simulink model "myexp6_2"  (R2022a)
settings: Solver=VariableStepAuto  StartTime=0.0  StopTime=10000  RelTol=1e-3
values from neighbouring files (symbols this model uses):
  Ns = Ns_list(i)    [exp6_1.m]
libraries: commsink2 x9, commchan3 x4, commrandsrc3 x4, dspsigops x4, dspstat3 x2
settings Model: Creator=惠普  LastModifiedBy=惠普

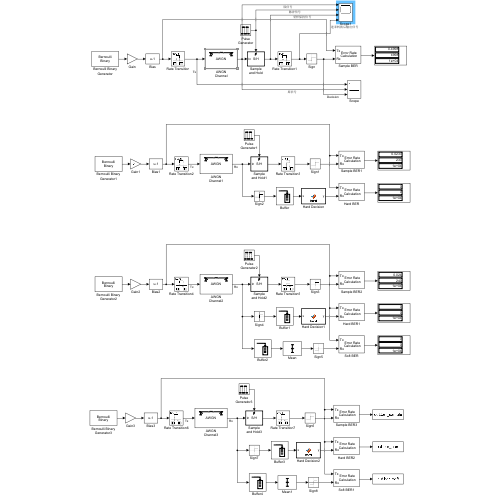
[thumbnail: Simulink's stored preview of the top-level diagram]
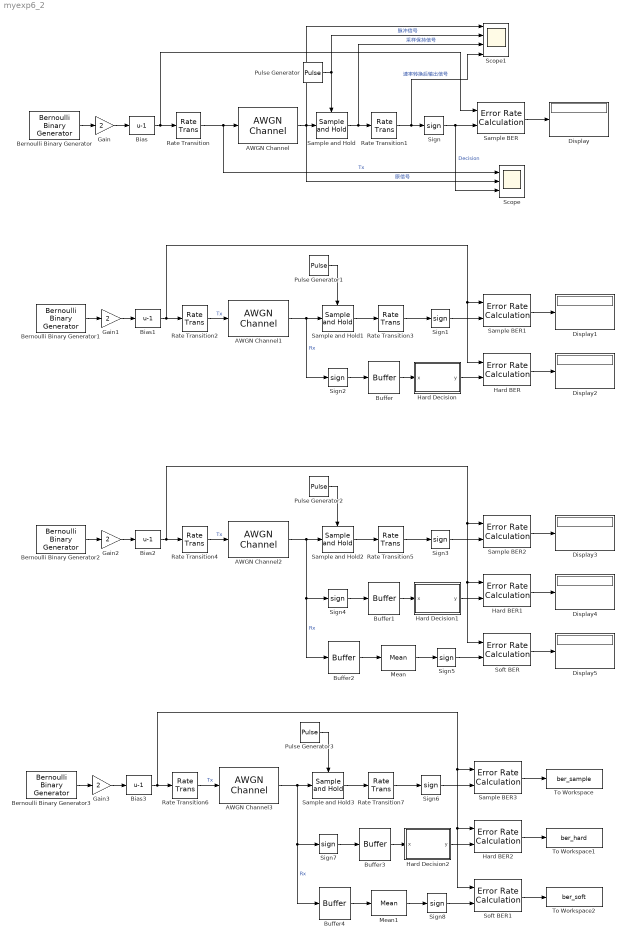
== system myexp6_2 ==
  AWGN Channel{,1..3} (4 alike) : commchan3/AWGN Channel  InputProcessing=Columns as channels (frame based)  seed=137  noiseMode=Variance from mask  EbNodB=10  EsNodB=10  SNRdB=10  bitsPerSym=1  Ps=1  Tsym=1  variance=sigma2
  Bernoulli Binary Generator{,1..3} (4 alike) : commrandsrc3/Bernoulli Binary Generator  ProbabilityOfZero=0.5  SeedSource=Auto  Seed=0  SampleTime=1  SamplesPerFrame=1  OutputDataType=double  SimulateUsing=Interpreted execution
  Bias{,1..3} (4 alike) : Bias  Bias=-1  SaturateOnIntegerOverflow=off
  Buffer{,1..4} (5 alike) : Buffer  N=Ns  OutputFrames=off
  Display{,1..5} (6 alike) : Display
  Gain{,1..3} (4 alike) : Gain  Gain=2
  Hard BER : commsink2/Error Rate Calculation  N=1  st_delay=0  cp_mode=Entire frame  subframe=[]  PMode=Port  WsName=ErrorVec  RsMode2=off  stop=off  numErr=100  maxBits=1e6
  Hard BER1 : commsink2/Error Rate Calculation  N=1  st_delay=0  cp_mode=Entire frame  subframe=[]  PMode=Port  WsName=ErrorVec  RsMode2=off  stop=off  numErr=100  maxBits=1e6
  Hard BER2 : commsink2/Error Rate Calculation  N=1  st_delay=0  cp_mode=Entire frame  subframe=[]  PMode=Port  WsName=ErrorVec  RsMode2=off  stop=off  numErr=100  maxBits=1e6
  Hard Decision : MATLAB Function  TreatAsAtomicUnit=on
  Hard Decision1 : MATLAB Function  TreatAsAtomicUnit=on
  Hard Decision2 : MATLAB Function  TreatAsAtomicUnit=on
  Mean : dspstat3/Mean  run=off  InputProcessing=Columns as channels (frame based)  reset_popup=None  directionMode=Each column  dimension=1  roiEnable=off  roiType=Rectangles  roiPortion=Entire ROI  roiOutput=Individual statistics for each ROI  roiFlag=off  roundingMode=Floor  overflowMode=off  outputDataTypeStr=Inherit: Same as accumulator  outputMin=[]  outputMax=[]  outputLastDataTypeStr=Inherit: Same as accumulator
  Mean1 : dspstat3/Mean  run=off  InputProcessing=Columns as channels (frame based)  reset_popup=None  directionMode=Each column  dimension=1  roiEnable=off  roiType=Rectangles  roiPortion=Entire ROI  roiOutput=Individual statistics for each ROI  roiFlag=off  roundingMode=Floor  overflowMode=off  outputDataTypeStr=Inherit: Same as accumulator  outputMin=[]  outputMax=[]  outputLastDataTypeStr=Inherit: Same as accumulator
  Pulse Generator : DiscretePulseGenerator  Period=Ns  PhaseDelay=5  SampleTime=1/Ns
  Pulse Generator1 : DiscretePulseGenerator  Period=Ns  SampleTime=1/Ns
  Pulse Generator2 : DiscretePulseGenerator  Period=Ns  SampleTime=1/Ns
  Pulse Generator3 : DiscretePulseGenerator  Period=Ns  SampleTime=1/Ns
  Rate Transition{,2,4,6} (4 alike) : RateTransition  Integrity=off  OutPortSampleTimeOpt=Multiple of input port sample time  OutPortSampleTimeMultiple=1/Ns
  Rate Transition{1,3,5,7} (4 alike) : RateTransition  OutPortSampleTimeOpt=Multiple of input port sample time  OutPortSampleTimeMultiple=Ns
  Sample and Hold{,1..3} (4 alike) : dspsigops/Sample and Hold  trig=Rising edge  initCond=0  latchinput=off
  Sample BER{,1..3} (4 alike) : commsink2/Error Rate Calculation  N=0  st_delay=0  cp_mode=Entire frame  subframe=[]  PMode=Port  WsName=ErrorVec  RsMode2=off  stop=off  numErr=100  maxBits=1e6
  Scope : Scope  NumInputPorts=3
  Scope1 : Scope  NumInputPorts=4
  Sign{,1..8} (9 alike) : Signum
  Soft BER : commsink2/Error Rate Calculation  N=1  st_delay=0  cp_mode=Entire frame  subframe=[]  PMode=Port  WsName=ErrorVec  RsMode2=off  stop=off  numErr=100  maxBits=1e6
  Soft BER1 : commsink2/Error Rate Calculation  N=1  st_delay=0  cp_mode=Entire frame  subframe=[]  PMode=Port  WsName=ErrorVec  RsMode2=off  stop=off  numErr=100  maxBits=1e6
  To Workspace : ToWorkspace  VariableName=ber_sample  SampleTime=-1
      settings: MaxDataPoints=1
  To Workspace1 : ToWorkspace  VariableName=ber_hard  SampleTime=-1
      settings: MaxDataPoints=1
  To Workspace2 : ToWorkspace  VariableName=ber_soft  SampleTime=-1
      settings: MaxDataPoints=1
  wires:
  Sample BER/1 -> Display/1
  Bernoulli Binary Generator/1 -> Gain/1
  Gain/1 -> Bias/1
  Sign/1 -> Scope/3, Sample BER/2  "Decision"
  AWGN Channel/1 -> Scope1/1, Sample and Hold/1, Scope/2  "原信号"
  Bias/1 -> Sample BER/1, Rate Transition/1
  Rate Transition/1 -> Scope/1, AWGN Channel/1  "Tx"
  Sample and Hold/1 -> Scope1/3, Rate Transition1/1  "采样保持信号"
  Rate Transition1/1 -> Scope1/4, Sign/1  "速率转换后输出信号"
  Pulse Generator/1 -> Sample and Hold/Trigger, Scope1/2  "脉冲信号"
  Rate Transition2/1 -> AWGN Channel1/1  "Tx"
  Rate Transition3/1 -> Sign1/1
  Bias1/1 -> Hard BER/1, Sample BER1/1, Rate Transition2/1
  Sample and Hold1/1 -> Rate Transition3/1
  Pulse Generator1/1 -> Sample and Hold1/Trigger
  Bernoulli Binary Generator1/1 -> Gain1/1
  Sample BER1/1 -> Display1/1
  AWGN Channel1/1 -> Sign2/1, Sample and Hold1/1  "Rx"
  Sign1/1 -> Sample BER1/2
  Gain1/1 -> Bias1/1
  Sign2/1 -> Buffer/1
  Hard BER/1 -> Display2/1
  Buffer/1 -> Hard Decision/1(x)
  Hard Decision/1(y) -> Hard BER/2
  Hard Decision1/1(y) -> Hard BER1/2
  Buffer1/1 -> Hard Decision1/1(x)
  Hard BER1/1 -> Display4/1
  AWGN Channel2/1 -> Buffer2/1, Sign4/1, Sample and Hold2/1  "Rx"
  Bernoulli Binary Generator2/1 -> Gain2/1
  Sample BER2/1 -> Display3/1
  Sign3/1 -> Sample BER2/2
  Bias2/1 -> Soft BER/1, Hard BER1/1, Sample BER2/1, Rate Transition4/1
  Rate Transition4/1 -> AWGN Channel2/1  "Tx"
  Rate Transition5/1 -> Sign3/1
  Pulse Generator2/1 -> Sample and Hold2/Trigger
  Sign4/1 -> Buffer1/1
  Gain2/1 -> Bias2/1
  Sample and Hold2/1 -> Rate Transition5/1
  Buffer2/1 -> Mean/1
  Mean/1 -> Sign5/1
  Soft BER/1 -> Display5/1
  Sign5/1 -> Soft BER/2
  Buffer4/1 -> Mean1/1
  Soft BER1/1 -> To Workspace2/1
  Gain3/1 -> Bias3/1
  Pulse Generator3/1 -> Sample and Hold3/Trigger
  Rate Transition7/1 -> Sign6/1
  Sample and Hold3/1 -> Rate Transition7/1
  Bernoulli Binary Generator3/1 -> Gain3/1
  Hard Decision2/1(y) -> Hard BER2/2
  Sign7/1 -> Buffer3/1
  Sign6/1 -> Sample BER3/2
  Bias3/1 -> Soft BER1/1, Hard BER2/1, Sample BER3/1, Rate Transition6/1
  Rate Transition6/1 -> AWGN Channel3/1  "Tx"
  Sample BER3/1 -> To Workspace/1
  Buffer3/1 -> Hard Decision2/1(x)
  Mean1/1 -> Sign8/1
  AWGN Channel3/1 -> Buffer4/1, Sign7/1, Sample and Hold3/1  "Rx"
  Hard BER2/1 -> To Workspace1/1
  Sign8/1 -> Soft BER1/2

== matlab function myexp6_2/Hard Decision ==
  data: x input; y output
function y = hard(x)
n0 = length(find(x==-1));
n1 = length(find(x==1));
if (n0>=n1)
    y = -1;
else
    y = 1;
end

== matlab function myexp6_2/Hard Decision2 ==
  data: x input; y output
function y = hard(x)
n0 = length(find(x==-1));
n1 = length(find(x==1));
if (n0>=n1)
    y = -1;
else
    y = 1;
end

== matlab function myexp6_2/Hard Decision1 ==
  data: x input; y output
function y = hard(x)
n0 = length(find(x==-1));
n1 = length(find(x==1));
if (n0>=n1)
    y = -1;
else
    y = 1;
end
